simulink model "tracking"  (R2022b)
settings: Solver=VariableStepAuto  StartTime=0.0  StopTime=100  RelTol=1e-3
libraries: robotmobilelib x1
settings Model: Creator=Admin  LastModifiedBy=Admin

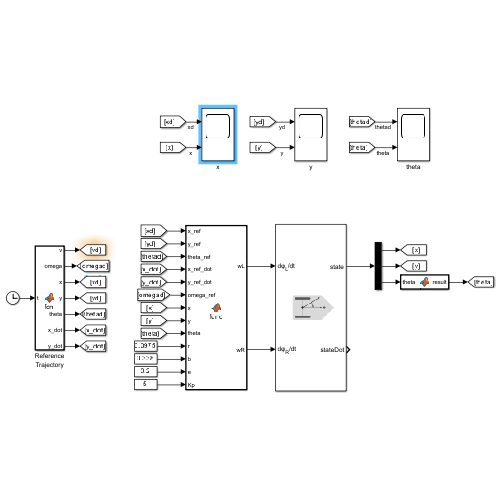
[thumbnail: Simulink's stored preview of the top-level diagram]
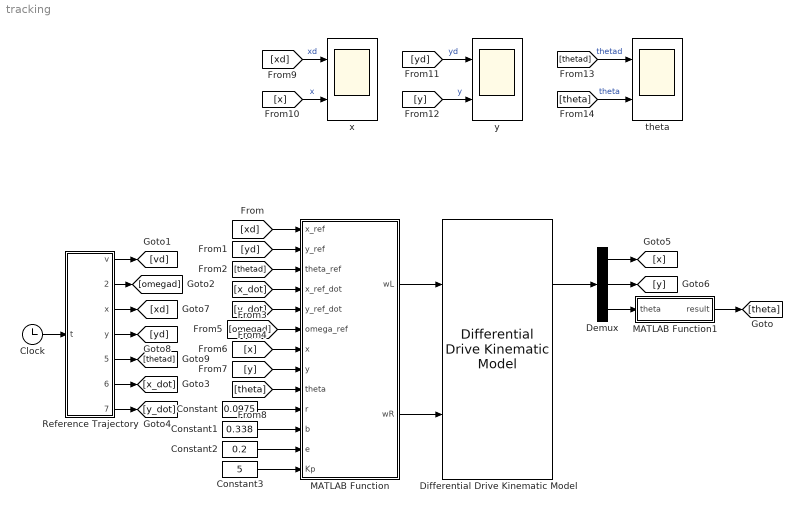
== system tracking ==
  Clock : Clock
  Constant : Constant  Value=0.0975
  Constant1 : Constant  Value=0.338
  Constant2 : Constant  Value=0.2
  Constant3 : Constant  Value=5
  Demux : Demux  Outputs=3
  Differential Drive Kinematic Model : robotmobilelib/Differential Drive Kinematic Model  VehicleInputs=Wheel Speeds  WheelRadius=0.0975  WheelSpeedRange=[-inf inf]  TrackWidth=0.338  InitialState=[0; 0; 0]  SimulateUsing=Interpreted execution
  MATLAB Function : MATLAB Function  TreatAsAtomicUnit=on
  MATLAB Function1 : MATLAB Function  TreatAsAtomicUnit=on
  Reference Trajectory : MATLAB Function  TreatAsAtomicUnit=on
  theta : Scope  NumInputPorts=2
  x : Scope  NumInputPorts=2
  y : Scope  NumInputPorts=2
  wires:
  Clock/1 -> Reference Trajectory/1(t)
  Reference Trajectory/2(omega) -> [omegad]
  Reference Trajectory/1(v) -> [vd]
  Reference Trajectory/3(x) -> [xd]
  Reference Trajectory/5(theta) -> [thetad]
  Reference Trajectory/4(y) -> [yd]
  Reference Trajectory/6(x_dot) -> [x_dot]
  Reference Trajectory/7(y_dot) -> [y_dot]
  [xd] -> MATLAB Function/1(x_ref)
  [yd] -> MATLAB Function/2(y_ref)
  [thetad] -> MATLAB Function/3(theta_ref)
  [x_dot] -> MATLAB Function/4(x_ref_dot)
  [y_dot] -> MATLAB Function/5(y_ref_dot)
  [omegad] -> MATLAB Function/6(omega_ref)
  MATLAB Function/1(wL) -> Differential Drive Kinematic Model/1
  MATLAB Function/2(wR) -> Differential Drive Kinematic Model/2
  Constant/1 -> MATLAB Function/10(r)
  Constant1/1 -> MATLAB Function/11(b)
  Constant2/1 -> MATLAB Function/12(e)
  Constant3/1 -> MATLAB Function/13(Kp)
  Differential Drive Kinematic Model/1 -> Demux/1
  Demux/1 -> [x]
  Demux/2 -> [y]
  Demux/3 -> MATLAB Function1/1(theta)
  [x] -> MATLAB Function/7(x)
  [y] -> MATLAB Function/8(y)
  [theta] -> MATLAB Function/9(theta)
  [xd] -> x/1  "xd"
  [x] -> x/2  "x"
  [yd] -> y/1  "yd"
  [y] -> y/2  "y"
  [thetad] -> theta/1  "thetad"
  [theta] -> theta/2  "theta"
  MATLAB Function1/1(result) -> [theta]

== matlab function tracking/MATLAB Function ==
  data: x_ref input; wL output; y_ref input; theta_ref input; x_ref_dot input; y_ref_dot input; omega_ref input; x input; y input; theta input; r input; b input; e input; Kp input; wR output
function [wL, wR] = func(x_ref, y_ref, theta_ref, x_ref_dot, y_ref_dot, omega_ref, x, y, theta, r, b, e, Kp)
wL = (((Kp * e ^ 2 - b * e * omega_ref) * cos(theta_ref) + (-Kp * b * e - e ^ 2 * omega_ref) * sin(theta_ref) + ((-x + x_ref) * Kp + x_ref_dot) * e - b * ((-y + y_ref) * Kp + y_ref_dot)) * cos(theta) + ((Kp * b * e + e ^ 2 * omega_ref) * cos(theta_ref) + (Kp * e ^ 2 - b * e * omega_ref) * sin(theta_ref) + ((-y + y_ref) * Kp + y_ref_dot) * e + b * ((-x + x_ref) * Kp + x_ref_dot)) * sin(theta) - Kp * e ^ 2) / r / e;
wR = (((Kp * e ^ 2 + b * e * omega_ref) * cos(theta_ref) + (Kp * b * e - e ^ 2 * omega_ref) * sin(theta_ref) + ((-x + x_ref) * Kp + x_ref_dot) * e + b * ((-y + y_ref) * Kp + y_ref_dot)) * cos(theta) + ((-Kp * b * e + e ^ 2 * omega_ref) * cos(theta_ref) + (Kp * e ^ 2 + b * e * omega_ref) * sin(theta_ref) + ((-y + y_ref) * Kp + y_ref_dot) * e - b * ((-x + x_ref) * Kp + x_ref_dot)) * sin(theta) - Kp * e ^ 2) / r / e;
end

== matlab function tracking/Reference Trajectory ==
  data: v output; omega output; x output; t input; y output; theta output; x_dot output; y_dot output
function [v, omega, x, y, theta, x_dot, y_dot] = fcn(t)
x = 0.1*sin(t);
y = 0.1*cos(t);
x_dot = 0.1*cos(t);
y_dot = -0.1*sin(t);
x_dotdot = -0.1*sin(t);
y_dotdot = -0.1*cos(t);
v = sqrt(x_dot^2 + y_dot^2);
theta = atan2(y_dot, x_dot);
omega = (x_dot*y_dotdot  - x_dotdot*y_dot)/(sqrt(x_dot^2 + y_dot^2));
end

== matlab function tracking/MATLAB Function1 ==
  data: theta input; result output
function result = fcn(theta)
result = mod(theta, 2*pi);
if (result > pi)
   result = result -2*pi;
end
if result < -pi
    result = 2*pi + result;
end
end
